simulink library "GFe_Lib"  (R2021a)
settings: Solver=VariableStepAuto  StartTime=0.0  StopTime=10.0  RelTol=1e-3
values from neighbouring files (symbols this model uses):
  Ki_i = 0    [Init_GFL.m]
  Kp_i = Lc_eq/wb*wn_i    [Init_GFL.m]
  Lf_pu = Lc_eq    [Init_GFL.m]
  Va0 = Vm0*sqrt(2)*Vb1*sin(Theta_Vm0*pi/180)    [Init_LF_L.m]    (also in Init_LF_MMC.m)
  Vb0 = Vm0*sqrt(2)*Vb1*sin(Theta_Vm0*pi/180-2*pi/3)    [Init_LF_L.m]    (also in Init_LF_MMC.m)
  Vc0 = Vm0*sqrt(2)*Vb1*sin(Theta_Vm0*pi/180+2*pi/3)    [Init_LF_L.m]    (also in Init_LF_MMC.m)
  Vm0_d = Vvsc0*cos(angle(Vvirt))    [Init_LF_L.m]    (also in Init_LF_MMC.m)
  Vm0_q = Vvsc0*sin(angle(Vvirt))    [Init_LF_L.m]    (also in Init_LF_MMC.m)
  Vvsc0 = abs(Vvirt)    [Init_LF_L.m]    (also in Init_LF_MMC.m)
undefined symbols (not defined in the file or in its folder): fb, Ib2, Sb, Solver_Time_Step, Time_Step, Vb1, Vb2, wb, Zb
libraries: Control_Lib x18, spsThreePhaseSourceLib x7, powerlib x7, spsThreePhaseBreakerLib x6, slpidlib x6, spsThreePhaseVIMeasurementLib x5, spsThreePhaseTransformerTwoWindingsLib x4, spsUniversalBridgeLib x3, spsVoltageMeasurementLib x3, spsRMSLib x2, spsDCVoltageSourceLib x2, spsSeriesRLCBranchLib x2
(part 3 of 3)

== system GFe_Lib/Mean Model 2-Level L-filter with DC Link/Control loops/ pu P//Q computation ==
  v_abc_pu : Inport  PortDimensions=3
  i_abc_pu : Inport  Port=2  PortDimensions=3
  Demux : Demux  Outputs=3
      settings: DisplayOption=none
  Mux : Mux  Inputs=3
  Product1 : Product  InputSameDT=on  SaturateOnIntegerOverflow=on  OutDataTypeStr=Inherit: Same as first input
  Product3 : Product  InputSameDT=on  SaturateOnIntegerOverflow=on  OutDataTypeStr=Inherit: Same as first input
  Sum : Sum  Inputs=+-  InputSameDT=on  SaturateOnIntegerOverflow=on  OutDataTypeStr=Inherit: Same as first input
  Sum1 : Sum  Inputs=1  InputSameDT=on  SaturateOnIntegerOverflow=on  OutDataTypeStr=Inherit: Same as first input
  Sum4 : Sum  Inputs=1  InputSameDT=on  SaturateOnIntegerOverflow=on  OutDataTypeStr=Inherit: Same as first input
  Sum5 : Sum  Inputs=+-  InputSameDT=on  SaturateOnIntegerOverflow=on  OutDataTypeStr=Inherit: Same as first input
  Sum6 : Sum  Inputs=+-  InputSameDT=on  SaturateOnIntegerOverflow=on  OutDataTypeStr=Inherit: Same as first input
  pu->V : Gain  Gain=1/sqrt(3)  SaturateOnIntegerOverflow=on  OutDataTypeStr=Inherit: Same as input  ParamDataTypeStr=Inherit: Same as input
  pu->V1 : Gain  Gain=1/3  SaturateOnIntegerOverflow=on  OutDataTypeStr=Inherit: Same as input  ParamDataTypeStr=Inherit: Same as input
  pu->V2 : Gain  Gain=1/3  SaturateOnIntegerOverflow=on  OutDataTypeStr=Inherit: Same as input  ParamDataTypeStr=Inherit: Same as input
  P : Outport  VectorParamsAs1DForOutWhenUnconnected=off
  Q : Outport  Port=2  VectorParamsAs1DForOutWhenUnconnected=off
  wires:
  pu->V/1 -> pu->V2/1  "Q"
  Mux/1 -> Product3/1
  Sum6/1 -> Mux/2
  Sum5/1 -> Mux/1
  Sum/1 -> Mux/3
  Demux/3 -> Sum6/1, Sum5/2
  Demux/2 -> Sum5/1, Sum/2
  Demux/1 -> Sum6/2, Sum/1
  Sum4/1 -> pu->V1/1
  i_abc_pu/1 -> Product3/2, Product1/2
  v_abc_pu/1 -> Demux/1, Product1/1
  Product1/1 -> Sum4/1
  Product3/1 -> Sum1/1
  Sum1/1 -> pu->V/1
  pu->V1/1 -> P/1
  pu->V2/1 -> Q/1

== system GFe_Lib/Mean Model 2-Level L-filter with DC Link/Control loops/Inner Current Control ==
  ig_dq_ref : Inport
  ig_dq : Inport  Port=2
  w_PLL : Inport  Port=3
  vg_dq : Inport  Port=4
  ig_dq_max : Inport  Port=5
  Current PI control : Subsystem
  vm_dq : Outport  VectorParamsAs1DForOutWhenUnconnected=off
  wires:
  w_PLL/1 -> Current PI control/4(w)  "w"
  vg_dq/1 -> Current PI control/2(Eg_dqfr)  "Eg_dq"
  ig_dq_ref/1 -> Current PI control/3(Is_dq_ref)
  Current PI control/1(vm_dq_ref) -> vm_dq/1  "vm_dq"
  ig_dq/1 -> Current PI control/1(Is_dq)  "Is_dq"
  ig_dq_max/1 -> Current PI control/5(Idq_ref_max)

== system GFe_Lib/Mean Model 2-Level L-filter with DC Link/Control loops/LPF ==
  In1 : Inport
  Add : Sum  Inputs=+-
  Gain : Gain  Gain=w_LPF
  Integrator : Integrator  InitialCondition=P0
  Out1 : Outport
  wires:
  In1/1 -> Add/1
  Integrator/1 -> Add/2, Out1/1
  Gain/1 -> Integrator/1
  Add/1 -> Gain/1

== system GFe_Lib/Mean Model 2-Level L-filter with DC Link/Control loops/LPF1 ==
  In1 : Inport
  Add : Sum  Inputs=+-
  Gain : Gain  Gain=w_LPF
  Integrator : Integrator  InitialCondition=V0
  Out1 : Outport
  wires:
  In1/1 -> Add/1
  Integrator/1 -> Add/2, Out1/1
  Gain/1 -> Integrator/1
  Add/1 -> Gain/1

== system GFe_Lib/Mean Model 2-Level L-filter with DC Link/Control loops/LPF2 ==
  In1 : Inport
  Add : Sum  Inputs=+-
  Gain : Gain  Gain=w_LPF
  Integrator : Integrator  InitialCondition=Q0
  Out1 : Outport
  wires:
  In1/1 -> Add/1
  Integrator/1 -> Add/2, Out1/1
  Gain/1 -> Integrator/1
  Add/1 -> Gain/1

== system GFe_Lib/Mean Model 2-Level L-filter with DC Link/Control loops/RMS derivation ==
  dq : Inport
  Demux : Demux  Outputs=2
  Sqrt : Sqrt  SaturateOnIntegerOverflow=on
  Square : Math  Operator=square  SaturateOnIntegerOverflow=on
  Square1 : Math  Operator=square  SaturateOnIntegerOverflow=on
  Sum : Sum
  rms : Outport
  wires:
  dq/1 -> Demux/1
  Demux/2 -> Square1/1
  Square/1 -> Sum/1
  Demux/1 -> Square/1
  Sqrt/1 -> rms/1
  Sum/1 -> Sqrt/1
  Square1/1 -> Sum/2

== system GFe_Lib/Mean Model 2-Level L-filter with DC Link/Control loops/norm1 ==
  In1 : Inport
  Add : Sum
  Demux : Demux  Outputs=2
  Sqrt : Sqrt  SaturateOnIntegerOverflow=on
  Square : Math  Operator=square  SaturateOnIntegerOverflow=on
  Square1 : Math  Operator=square  SaturateOnIntegerOverflow=on
  Out1 : Outport
  wires:
  In1/1 -> Demux/1
  Square1/1 -> Add/2
  Square/1 -> Add/1
  Demux/1 -> Square/1
  Demux/2 -> Square1/1
  Add/1 -> Sqrt/1
  Sqrt/1 -> Out1/1

== system GFe_Lib/Mean Model 2-Level L-filter with DC Link/Control loops/norm2 ==
  In1 : Inport
  Add : Sum
  Demux : Demux  Outputs=2
  Sqrt : Sqrt  SaturateOnIntegerOverflow=on
  Square : Math  Operator=square  SaturateOnIntegerOverflow=on
  Square1 : Math  Operator=square  SaturateOnIntegerOverflow=on
  Out1 : Outport
  wires:
  In1/1 -> Demux/1
  Square1/1 -> Add/2
  Square/1 -> Add/1
  Demux/1 -> Square/1
  Demux/2 -> Square1/1
  Add/1 -> Sqrt/1
  Sqrt/1 -> Out1/1

== system GFe_Lib/Mean Model 2-Level L-filter_sav/Control loops/ pu P//Q computation ==
  v_abc_pu : Inport  PortDimensions=3
  i_abc_pu : Inport  Port=2  PortDimensions=3
  Demux : Demux  Outputs=3
      settings: DisplayOption=none
  Mux : Mux  Inputs=3
  Product1 : Product  InputSameDT=on  SaturateOnIntegerOverflow=on  OutDataTypeStr=Inherit: Same as first input
  Product3 : Product  InputSameDT=on  SaturateOnIntegerOverflow=on  OutDataTypeStr=Inherit: Same as first input
  Sum : Sum  Inputs=+-  InputSameDT=on  SaturateOnIntegerOverflow=on  OutDataTypeStr=Inherit: Same as first input
  Sum1 : Sum  Inputs=1  InputSameDT=on  SaturateOnIntegerOverflow=on  OutDataTypeStr=Inherit: Same as first input
  Sum4 : Sum  Inputs=1  InputSameDT=on  SaturateOnIntegerOverflow=on  OutDataTypeStr=Inherit: Same as first input
  Sum5 : Sum  Inputs=+-  InputSameDT=on  SaturateOnIntegerOverflow=on  OutDataTypeStr=Inherit: Same as first input
  Sum6 : Sum  Inputs=+-  InputSameDT=on  SaturateOnIntegerOverflow=on  OutDataTypeStr=Inherit: Same as first input
  pu->V : Gain  Gain=1/sqrt(3)  SaturateOnIntegerOverflow=on  OutDataTypeStr=Inherit: Same as input  ParamDataTypeStr=Inherit: Same as input
  pu->V1 : Gain  Gain=1/3  SaturateOnIntegerOverflow=on  OutDataTypeStr=Inherit: Same as input  ParamDataTypeStr=Inherit: Same as input
  pu->V2 : Gain  Gain=1/3  SaturateOnIntegerOverflow=on  OutDataTypeStr=Inherit: Same as input  ParamDataTypeStr=Inherit: Same as input
  P : Outport  VectorParamsAs1DForOutWhenUnconnected=off
  Q : Outport  Port=2  VectorParamsAs1DForOutWhenUnconnected=off
  wires:
  pu->V2/1 -> Q/1
  pu->V1/1 -> P/1
  Sum1/1 -> pu->V/1
  Product3/1 -> Sum1/1
  Product1/1 -> Sum4/1
  v_abc_pu/1 -> Product1/1, Demux/1
  i_abc_pu/1 -> Product1/2, Product3/2
  Sum4/1 -> pu->V1/1
  Demux/1 -> Sum/1, Sum6/2
  Demux/2 -> Sum/2, Sum5/1
  Demux/3 -> Sum5/2, Sum6/1
  Sum/1 -> Mux/3
  Sum5/1 -> Mux/1
  Sum6/1 -> Mux/2
  Mux/1 -> Product3/1
  pu->V/1 -> pu->V2/1  "Q"

== system GFe_Lib/Mean Model 2-Level L-filter_sav/Control loops/Inner Current Control ==
  ig_dq_ref : Inport
  ig_dq : Inport  Port=2
  theta_PLL : Inport  Port=3
  w_PLL : Inport  Port=4
  vg_dq : Inport  Port=5
  Control Delay compensation : Constant  Value=wb*Solver_Time_Step
  Current PI control : Subsystem
  Mux : Mux  Inputs=2
  Sum : Sum  Inputs=|++
  Trigonometric Function : Trigonometry
  Trigonometric Function1 : Trigonometry  Operator=cos
  vm_dq : Outport  VectorParamsAs1DForOutWhenUnconnected=off
  CosSinTheta_delay : Outport  Port=2  VectorParamsAs1DForOutWhenUnconnected=off
  wires:
  ig_dq/1 -> Current PI control/1(Is_dq)  "Is_dq"
  Current PI control/1(vm_dq_ref) -> vm_dq/1  "vm_dq"
  ig_dq_ref/1 -> Current PI control/3(Is_dq_ref)
  vg_dq/1 -> Current PI control/2(Eg_dqfr)  "Eg_dq"
  w_PLL/1 -> Current PI control/4(w)  "w"
  Control Delay compensation/1 -> Sum/2
  Trigonometric Function/1 -> Mux/2
  Sum/1 -> Trigonometric Function/1, Trigonometric Function1/1
  theta_PLL/1 -> Sum/1  "Theta"
  Trigonometric Function1/1 -> Mux/1
  Mux/1 -> CosSinTheta_delay/1

== system GFe_Lib/Mean Model 2-Level LCL-filter [under construction]/Control loops/ pu P//Q computation ==
  v_abc_pu : Inport  PortDimensions=3
  i_abc_pu : Inport  Port=2  PortDimensions=3
  Demux : Demux  Outputs=3
      settings: DisplayOption=none
  Mux : Mux  Inputs=3
  Product1 : Product  InputSameDT=on  SaturateOnIntegerOverflow=on  OutDataTypeStr=Inherit: Same as first input
  Product3 : Product  InputSameDT=on  SaturateOnIntegerOverflow=on  OutDataTypeStr=Inherit: Same as first input
  Sum : Sum  Inputs=+-  InputSameDT=on  SaturateOnIntegerOverflow=on  OutDataTypeStr=Inherit: Same as first input
  Sum1 : Sum  Inputs=1  InputSameDT=on  SaturateOnIntegerOverflow=on  OutDataTypeStr=Inherit: Same as first input
  Sum4 : Sum  Inputs=1  InputSameDT=on  SaturateOnIntegerOverflow=on  OutDataTypeStr=Inherit: Same as first input
  Sum5 : Sum  Inputs=+-  InputSameDT=on  SaturateOnIntegerOverflow=on  OutDataTypeStr=Inherit: Same as first input
  Sum6 : Sum  Inputs=+-  InputSameDT=on  SaturateOnIntegerOverflow=on  OutDataTypeStr=Inherit: Same as first input
  pu->V : Gain  Gain=1/sqrt(3)  SaturateOnIntegerOverflow=on  OutDataTypeStr=Inherit: Same as input  ParamDataTypeStr=Inherit: Same as input
  pu->V1 : Gain  Gain=1/3  SaturateOnIntegerOverflow=on  OutDataTypeStr=Inherit: Same as input  ParamDataTypeStr=Inherit: Same as input
  pu->V2 : Gain  Gain=1/3  SaturateOnIntegerOverflow=on  OutDataTypeStr=Inherit: Same as input  ParamDataTypeStr=Inherit: Same as input
  P : Outport  VectorParamsAs1DForOutWhenUnconnected=off
  Q : Outport  Port=2  VectorParamsAs1DForOutWhenUnconnected=off
  wires:
  pu->V2/1 -> Q/1
  pu->V1/1 -> P/1
  Sum1/1 -> pu->V/1
  Product3/1 -> Sum1/1
  Product1/1 -> Sum4/1
  v_abc_pu/1 -> Product1/1, Demux/1
  i_abc_pu/1 -> Product1/2, Product3/2
  Sum4/1 -> pu->V1/1
  Demux/1 -> Sum/1, Sum6/2
  Demux/2 -> Sum/2, Sum5/1
  Demux/3 -> Sum5/2, Sum6/1
  Sum/1 -> Mux/3
  Sum5/1 -> Mux/1
  Sum6/1 -> Mux/2
  Mux/1 -> Product3/1
  pu->V/1 -> pu->V2/1  "Q"

== system GFe_Lib/Mean Model 2-Level LCL-filter [under construction]/Control loops/Inner Current Control ==
  ig_dq_ref : Inport
  ig_dq : Inport  Port=2
  theta_PLL : Inport  Port=3
  w_PLL : Inport  Port=4
  vg_dq : Inport  Port=5
  Current PI control : Subsystem
  vm_dq : Outport  VectorParamsAs1DForOutWhenUnconnected=off
  theta : Outport  Port=2  VectorParamsAs1DForOutWhenUnconnected=off
  wires:
  ig_dq/1 -> Current PI control/1(Is_dq)  "Is_dq"
  theta_PLL/1 -> theta/1  "Theta"
  Current PI control/1(vm_dq_ref) -> vm_dq/1  "vm_dq"
  ig_dq_ref/1 -> Current PI control/3(Is_dq_ref)
  vg_dq/1 -> Current PI control/2(Eg_dqfr)  "Eg_dq"
  w_PLL/1 -> Current PI control/4(w)  "w"

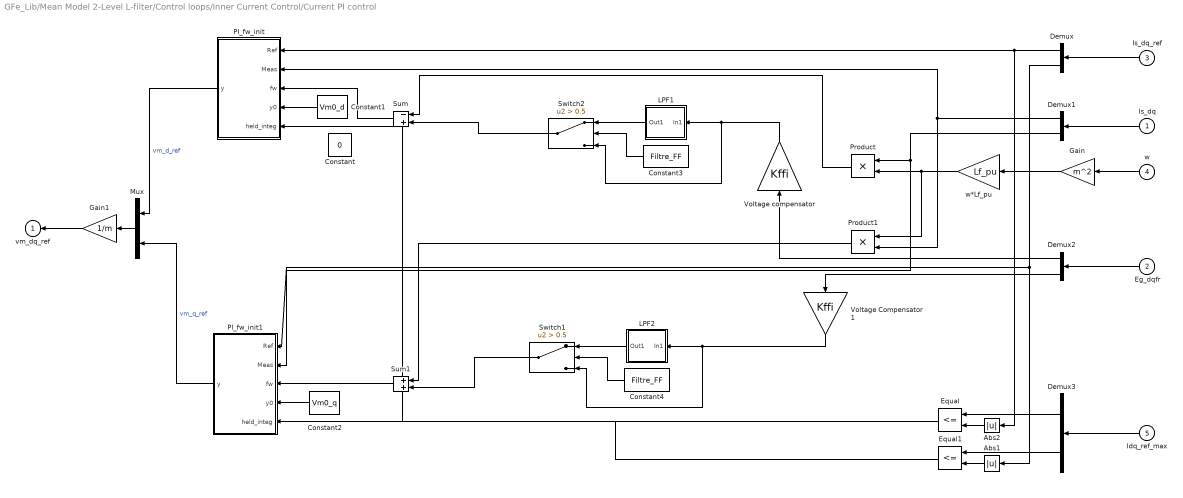
== system GFe_Lib/Mean Model 2-Level L-filter/Control loops/Inner Current Control/Current PI control ==
  Is_dq : Inport
  Eg_dqfr : Inport  Port=2
  Is_dq_ref : Inport  Port=3
  w : Inport  Port=4
  Idq_ref_max : Inport  Port=5
  Abs1 : Abs
  Abs2 : Abs
  Constant : Constant  Value=0
  Constant1 : Constant  Value=Vm0_d
  Constant2 : Constant  Value=Vm0_q
  Constant3 : Constant  Value=Filtre_FF
  Constant4 : Constant  Value=Filtre_FF
  Demux{,1..3} (4 alike) : Demux  Outputs=2
  Equal : RelationalOperator  Operator=<=  OutDataTypeStr=boolean  RndMeth=Simplest
  Equal1 : RelationalOperator  Operator=<=  OutDataTypeStr=boolean  RndMeth=Simplest
  Gain : Gain  Gain=m^2
  Gain1 : Gain  Gain=1/m
  LPF1 : Subsystem
  LPF2 : Subsystem
  Mux : Mux  Inputs=[1 1]
  PI_fw_init : Subsystem  AncestorBlock=Control_Lib/PI_fw_init  TreatAsAtomicUnit=on  mask{Kp=Kp_i, Ki=Ki_i}
  PI_fw_init1 : Subsystem  AncestorBlock=Control_Lib/PI_fw_init  TreatAsAtomicUnit=on  mask{Kp=Kp_i, Ki=Ki_i}
  Product : Product  RndMeth=Zero
  Product1 : Product  RndMeth=Zero
  Sum : Sum  Inputs=-+
  Sum1 : Sum
  Switch1 : Switch  Criteria=u2 > Threshold  Threshold=0.5
  Switch2 : Switch  Criteria=u2 > Threshold  Threshold=0.5
  Voltage Compensator 1 : Gain  Gain=Kffi
  Voltage compensator : Gain  Gain=Kffi
  w*Lf_pu : Gain  Gain=Lf_pu
  vm_dq_ref : Outport  InitialOutput=0  VectorParamsAs1DForOutWhenUnconnected=off
  wires:
  Voltage compensator/1 -> Switch2/3, LPF1/1(In1)
  w/1 -> Gain/1
  PI_fw_init1/1(y) -> Mux/2  "vm_q_ref"
  PI_fw_init/1(y) -> Mux/1  "vm_d_ref"
  Product1/1 -> Sum1/1
  Demux/2 -> Abs1/1, PI_fw_init1/1(Ref)
  Mux/1 -> Gain1/1
  Demux1/2 -> PI_fw_init1/2(Meas), Product/1
  w*Lf_pu/1 -> Product/2, Product1/1
  Demux1/1 -> PI_fw_init/2(Meas), Product1/2
  Demux/1 -> PI_fw_init/1(Ref), Abs2/1
  Is_dq_ref/1 -> Demux/1
  Is_dq/1 -> Demux1/1
  Eg_dqfr/1 -> Demux2/1
  Product/1 -> Sum/1
  Sum/1 -> PI_fw_init/3(fw)
  Constant1/1 -> PI_fw_init/4(y0)
  Sum1/1 -> PI_fw_init1/3(fw)
  Constant2/1 -> PI_fw_init1/4(y0)
  Demux2/1 -> Voltage compensator/1
  Demux2/2 -> Voltage Compensator 1/1
  Idq_ref_max/1 -> Demux3/1
  Demux3/1 -> Equal/1
  Demux3/2 -> Equal1/1
  Abs2/1 -> Equal/2
  Abs1/1 -> Equal1/2
  Equal/1 -> PI_fw_init/5(held_integ)
  Equal1/1 -> PI_fw_init1/5(held_integ)
  Gain/1 -> w*Lf_pu/1
  Gain1/1 -> vm_dq_ref/1
  LPF1/1(Out1) -> Switch2/1
  Constant3/1 -> Switch2/2
  Switch2/1 -> Sum/2
  LPF2/1(Out1) -> Switch1/1
  Voltage Compensator 1/1 -> Switch1/3, LPF2/1(In1)
  Constant4/1 -> Switch1/2
  Switch1/1 -> Sum1/2

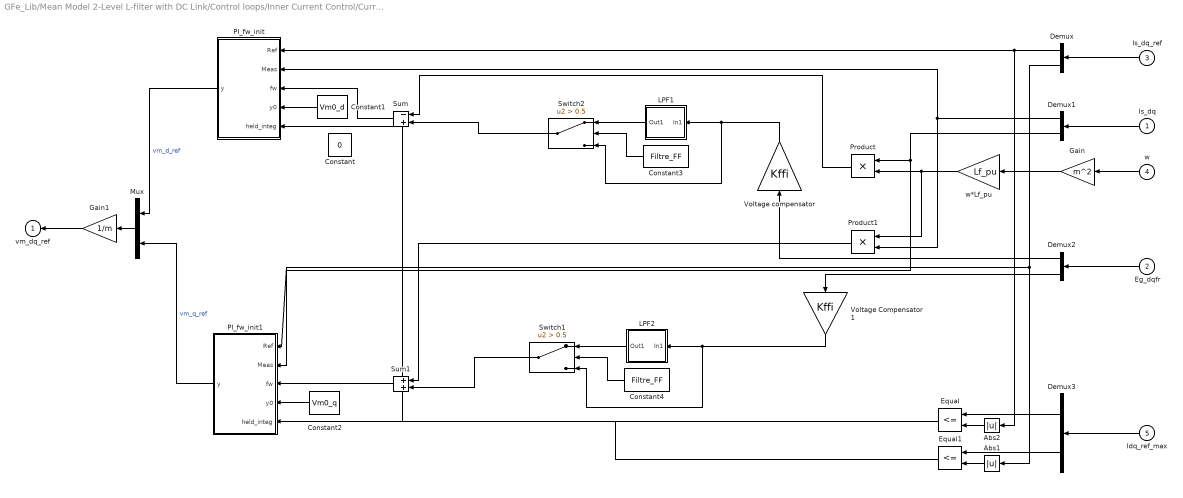
== system GFe_Lib/Mean Model 2-Level L-filter with DC Link/Control loops/Inner Current Control/Current PI control ==
  Is_dq : Inport
  Eg_dqfr : Inport  Port=2
  Is_dq_ref : Inport  Port=3
  w : Inport  Port=4
  Idq_ref_max : Inport  Port=5
  Abs1 : Abs
  Abs2 : Abs
  Constant : Constant  Value=0
  Constant1 : Constant  Value=Vm0_d
  Constant2 : Constant  Value=Vm0_q
  Constant3 : Constant  Value=Filtre_FF
  Constant4 : Constant  Value=Filtre_FF
  Demux{,1..3} (4 alike) : Demux  Outputs=2
  Equal : RelationalOperator  Operator=<=  OutDataTypeStr=boolean  RndMeth=Simplest
  Equal1 : RelationalOperator  Operator=<=  OutDataTypeStr=boolean  RndMeth=Simplest
  Gain : Gain  Gain=m^2
  Gain1 : Gain  Gain=1/m
  LPF1 : Subsystem
  LPF2 : Subsystem
  Mux : Mux  Inputs=[1 1]
  PI_fw_init : Subsystem  AncestorBlock=Control_Lib/PI_fw_init  TreatAsAtomicUnit=on  mask{Kp=Kp_i, Ki=Ki_i}
  PI_fw_init1 : Subsystem  AncestorBlock=Control_Lib/PI_fw_init  TreatAsAtomicUnit=on  mask{Kp=Kp_i, Ki=Ki_i}
  Product : Product  RndMeth=Zero
  Product1 : Product  RndMeth=Zero
  Sum : Sum  Inputs=-+
  Sum1 : Sum
  Switch1 : Switch  Criteria=u2 > Threshold  Threshold=0.5
  Switch2 : Switch  Criteria=u2 > Threshold  Threshold=0.5
  Voltage Compensator 1 : Gain  Gain=Kffi
  Voltage compensator : Gain  Gain=Kffi
  w*Lf_pu : Gain  Gain=Lf_pu
  vm_dq_ref : Outport  InitialOutput=0  VectorParamsAs1DForOutWhenUnconnected=off
  wires:
  Voltage compensator/1 -> Switch2/3, LPF1/1(In1)
  w/1 -> Gain/1
  PI_fw_init1/1(y) -> Mux/2  "vm_q_ref"
  PI_fw_init/1(y) -> Mux/1  "vm_d_ref"
  Product1/1 -> Sum1/1
  Demux/2 -> Abs1/1, PI_fw_init1/1(Ref)
  Mux/1 -> Gain1/1
  Demux1/2 -> PI_fw_init1/2(Meas), Product/1
  w*Lf_pu/1 -> Product/2, Product1/1
  Demux1/1 -> PI_fw_init/2(Meas), Product1/2
  Demux/1 -> PI_fw_init/1(Ref), Abs2/1
  Is_dq_ref/1 -> Demux/1
  Is_dq/1 -> Demux1/1
  Eg_dqfr/1 -> Demux2/1
  Product/1 -> Sum/1
  Sum/1 -> PI_fw_init/3(fw)
  Constant1/1 -> PI_fw_init/4(y0)
  Sum1/1 -> PI_fw_init1/3(fw)
  Constant2/1 -> PI_fw_init1/4(y0)
  Demux2/1 -> Voltage compensator/1
  Demux2/2 -> Voltage Compensator 1/1
  Idq_ref_max/1 -> Demux3/1
  Demux3/1 -> Equal/1
  Demux3/2 -> Equal1/1
  Abs2/1 -> Equal/2
  Abs1/1 -> Equal1/2
  Equal/1 -> PI_fw_init/5(held_integ)
  Equal1/1 -> PI_fw_init1/5(held_integ)
  Gain/1 -> w*Lf_pu/1
  Gain1/1 -> vm_dq_ref/1
  LPF1/1(Out1) -> Switch2/1
  Constant3/1 -> Switch2/2
  Switch2/1 -> Sum/2
  LPF2/1(Out1) -> Switch1/1
  Voltage Compensator 1/1 -> Switch1/3, LPF2/1(In1)
  Constant4/1 -> Switch1/2
  Switch1/1 -> Sum1/2

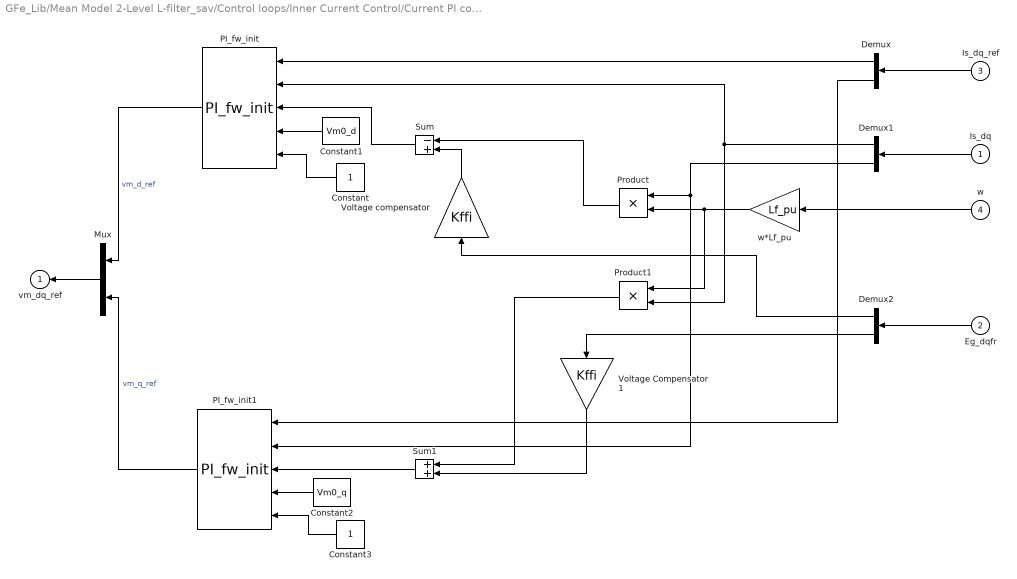
== system GFe_Lib/Mean Model 2-Level L-filter_sav/Control loops/Inner Current Control/Current PI control ==
  Is_dq : Inport
  Eg_dqfr : Inport  Port=2
  Is_dq_ref : Inport  Port=3
  w : Inport  Port=4
  Constant : Constant
  Constant1 : Constant  Value=Vm0_d
  Constant2 : Constant  Value=Vm0_q
  Constant3 : Constant
  Demux : Demux  Outputs=2
  Demux1 : Demux  Outputs=2
  Demux2 : Demux  Outputs=2
  Mux : Mux  Inputs=[1 1]
  PI_fw_init : Control_Lib/PI_fw_init  Kp=Kp_i  Ki=Ki_i
      settings: SourceProductName=VSC4SPS
  PI_fw_init1 : Control_Lib/PI_fw_init  Kp=Kp_i  Ki=Ki_i
      settings: SourceProductName=VSC4SPS
  Product : Product  RndMeth=Zero
  Product1 : Product  RndMeth=Zero
  Sum : Sum  Inputs=-+
  Sum1 : Sum
  Voltage Compensator 1 : Gain  Gain=Kffi
  Voltage compensator : Gain  Gain=Kffi
  w*Lf_pu : Gain  Gain=Lf_pu
  vm_dq_ref : Outport  InitialOutput=0  VectorParamsAs1DForOutWhenUnconnected=off
  wires:
  Constant3/1 -> PI_fw_init1/5
  Constant2/1 -> PI_fw_init1/4
  Voltage Compensator 1/1 -> Sum1/2
  Sum1/1 -> PI_fw_init1/3
  Constant1/1 -> PI_fw_init/4
  Constant/1 -> PI_fw_init/5
  Sum/1 -> PI_fw_init/3
  Product/1 -> Sum/1
  Eg_dqfr/1 -> Demux2/1
  Demux2/2 -> Voltage Compensator 1/1
  Demux2/1 -> Voltage compensator/1
  Is_dq/1 -> Demux1/1
  Is_dq_ref/1 -> Demux/1
  Demux/1 -> PI_fw_init/1
  Demux1/1 -> Product1/2, PI_fw_init/2
  w*Lf_pu/1 -> Product1/1, Product/2
  Demux1/2 -> Product/1, PI_fw_init1/2
  Mux/1 -> vm_dq_ref/1
  Demux/2 -> PI_fw_init1/1
  Product1/1 -> Sum1/1
  PI_fw_init/1 -> Mux/1  "vm_d_ref"
  PI_fw_init1/1 -> Mux/2  "vm_q_ref"
  w/1 -> w*Lf_pu/1
  Voltage compensator/1 -> Sum/2

== system GFe_Lib/Mean Model 2-Level LCL-filter [under construction]/Control loops/Inner Current Control/Current PI control ==
  Is_dq : Inport
  Eg_dqfr : Inport  Port=2
  Is_dq_ref : Inport  Port=3
  w : Inport  Port=4
  Constant : Constant
  Constant1 : Constant  Value=Vm0_d
  Constant2 : Constant  Value=Vm0_q
  Constant3 : Constant
  Demux : Demux  Outputs=2
  Demux1 : Demux  Outputs=2
  Demux2 : Demux  Outputs=2
  Mux : Mux  Inputs=[1 1]
  PI_fw_init : Control_Lib/PI_fw_init  Kp=Kp_i  Ki=Ki_i
      settings: SourceProductName=VSC4SPS
  PI_fw_init1 : Control_Lib/PI_fw_init  Kp=Kp_i  Ki=Ki_i
      settings: SourceProductName=VSC4SPS
  Product : Product  RndMeth=Zero
  Product1 : Product  RndMeth=Zero
  Sum : Sum  Inputs=-+
  Sum1 : Sum
  Voltage Compensator 1 : Gain  Gain=Kffi
  Voltage compensator : Gain  Gain=Kffi
  w*Lf_pu : Gain  Gain=Lf_pu
  vm_dq_ref : Outport  InitialOutput=0  VectorParamsAs1DForOutWhenUnconnected=off
  wires:
  Constant3/1 -> PI_fw_init1/5
  Constant2/1 -> PI_fw_init1/4
  Voltage Compensator 1/1 -> Sum1/2
  Sum1/1 -> PI_fw_init1/3
  Constant1/1 -> PI_fw_init/4
  Constant/1 -> PI_fw_init/5
  Sum/1 -> PI_fw_init/3
  Product/1 -> Sum/1
  Eg_dqfr/1 -> Demux2/1
  Demux2/2 -> Voltage Compensator 1/1
  Demux2/1 -> Voltage compensator/1
  Is_dq/1 -> Demux1/1
  Is_dq_ref/1 -> Demux/1
  Demux/1 -> PI_fw_init/1
  Demux1/1 -> Product1/2, PI_fw_init/2
  w*Lf_pu/1 -> Product1/1, Product/2
  Demux1/2 -> Product/1, PI_fw_init1/2
  Mux/1 -> vm_dq_ref/1
  Demux/2 -> PI_fw_init1/1
  Product1/1 -> Sum1/1
  PI_fw_init/1 -> Mux/1  "vm_d_ref"
  PI_fw_init1/1 -> Mux/2  "vm_q_ref"
  w/1 -> w*Lf_pu/1
  Voltage compensator/1 -> Sum/2

== system GFe_Lib/Mean Model 2-Level L-filter/Control loops/Inner Current Control/Current PI control/LPF1 ==
  In1 : Inport
  Add : Sum  Inputs=+-
  Gain : Gain  Gain=w_ff
  Integrator : Integrator  InitialCondition=V0*cos(Theta0*pi/180)
  Out1 : Outport
  wires:
  In1/1 -> Add/1
  Integrator/1 -> Add/2, Out1/1
  Gain/1 -> Integrator/1
  Add/1 -> Gain/1

== system GFe_Lib/Mean Model 2-Level L-filter/Control loops/Inner Current Control/Current PI control/LPF2 ==
  In1 : Inport
  Add : Sum  Inputs=+-
  Gain : Gain  Gain=w_ff
  Integrator : Integrator  InitialCondition=V0*sin(Theta0*pi/180)
  Out1 : Outport
  wires:
  In1/1 -> Add/1
  Integrator/1 -> Add/2, Out1/1
  Gain/1 -> Integrator/1
  Add/1 -> Gain/1

== system GFe_Lib/Mean Model 2-Level L-filter/Control loops/Inner Current Control/Current PI control/PI_fw_init ==
  Ref : Inport
  Meas : Inport  Port=2
  fw : Inport  Port=3
  y0 : Inport  Port=4
  held_integ : Inport  Port=5
  Constant : Constant  Value=0
  Constant1 : Constant  Value=0
  Data Type Conversion : DataTypeConversion
  Gain : Gain  Gain=Kp
  Gain1 : Gain  Gain=Ki
  Init_condition : Subsystem
  Integrator : Integrator  InitialConditionSource=external
  Memory : Memory  InitialCondition=1
  Subsystem : Subsystem  Commented=on
  Sum : Sum
  Sum1 : Sum  Inputs=+-
  Sum2 : Sum
  Switch : Switch  Criteria=u2 > Threshold  Threshold=0.5
  y : Outport  VectorParamsAs1DForOutWhenUnconnected=off
  wires:
  Init_condition/1(integ0) -> Integrator/2
  [comp] -> Init_condition/2(comp)
  Ref/1 -> Sum1/1
  Meas/1 -> Sum1/2
  Sum/1 -> Sum2/1, [comp]
  Sum1/1 -> Gain/1, Gain1/1
  Sum2/1 -> y/1
  y0/1 -> Init_condition/1(y0)
  Constant/1 -> Memory/1
  Memory/1 -> Init_condition/Enable
  fw/1 -> Sum/1
  Gain/1 -> Sum/2
  Integrator/1 -> Sum2/2
  Switch/1 -> Integrator/1
  Constant1/1 -> Switch/1
  Gain1/1 -> Switch/3
  held_integ/1 -> Data Type Conversion/1
  Data Type Conversion/1 -> Switch/2

== system GFe_Lib/Mean Model 2-Level L-filter/Control loops/Inner Current Control/Current PI control/PI_fw_init1 ==
  Ref : Inport
  Meas : Inport  Port=2
  fw : Inport  Port=3
  y0 : Inport  Port=4
  held_integ : Inport  Port=5
  Constant : Constant  Value=0
  Constant1 : Constant  Value=0
  Data Type Conversion : DataTypeConversion
  Gain : Gain  Gain=Kp
  Gain1 : Gain  Gain=Ki
  Init_condition : Subsystem
  Integrator : Integrator  InitialConditionSource=external
  Memory : Memory  InitialCondition=1
  Subsystem : Subsystem  Commented=on
  Sum : Sum
  Sum1 : Sum  Inputs=+-
  Sum2 : Sum
  Switch : Switch  Criteria=u2 > Threshold  Threshold=0.5
  y : Outport  VectorParamsAs1DForOutWhenUnconnected=off
  wires:
  Init_condition/1(integ0) -> Integrator/2
  [comp] -> Init_condition/2(comp)
  Ref/1 -> Sum1/1
  Meas/1 -> Sum1/2
  Sum/1 -> Sum2/1, [comp]
  Sum1/1 -> Gain/1, Gain1/1
  Sum2/1 -> y/1
  y0/1 -> Init_condition/1(y0)
  Constant/1 -> Memory/1
  Memory/1 -> Init_condition/Enable
  fw/1 -> Sum/1
  Gain/1 -> Sum/2
  Integrator/1 -> Sum2/2
  Switch/1 -> Integrator/1
  Constant1/1 -> Switch/1
  Gain1/1 -> Switch/3
  held_integ/1 -> Data Type Conversion/1
  Data Type Conversion/1 -> Switch/2

== system GFe_Lib/Mean Model 2-Level L-filter with DC Link/Control loops/Inner Current Control/Current PI control/LPF1 ==
  In1 : Inport
  Add : Sum  Inputs=+-
  Gain : Gain  Gain=w_ff
  Integrator : Integrator  InitialCondition=V0*cos(Theta0*pi/180)
  Out1 : Outport
  wires:
  In1/1 -> Add/1
  Integrator/1 -> Add/2, Out1/1
  Gain/1 -> Integrator/1
  Add/1 -> Gain/1

== system GFe_Lib/Mean Model 2-Level L-filter with DC Link/Control loops/Inner Current Control/Current PI control/LPF2 ==
  In1 : Inport
  Add : Sum  Inputs=+-
  Gain : Gain  Gain=w_ff
  Integrator : Integrator  InitialCondition=V0*sin(Theta0*pi/180)
  Out1 : Outport
  wires:
  In1/1 -> Add/1
  Integrator/1 -> Add/2, Out1/1
  Gain/1 -> Integrator/1
  Add/1 -> Gain/1

== system GFe_Lib/Mean Model 2-Level L-filter with DC Link/Control loops/Inner Current Control/Current PI control/PI_fw_init ==
  Ref : Inport
  Meas : Inport  Port=2
  fw : Inport  Port=3
  y0 : Inport  Port=4
  held_integ : Inport  Port=5
  Constant : Constant  Value=0
  Constant1 : Constant  Value=0
  Data Type Conversion : DataTypeConversion
  Gain : Gain  Gain=Kp
  Gain1 : Gain  Gain=Ki
  Init_condition : Subsystem
  Integrator : Integrator  InitialConditionSource=external
  Memory : Memory  InitialCondition=1
  Subsystem : Subsystem  Commented=on
  Sum : Sum
  Sum1 : Sum  Inputs=+-
  Sum2 : Sum
  Switch : Switch  Criteria=u2 > Threshold  Threshold=0.5
  y : Outport  VectorParamsAs1DForOutWhenUnconnected=off
  wires:
  Init_condition/1(integ0) -> Integrator/2
  [comp] -> Init_condition/2(comp)
  Ref/1 -> Sum1/1
  Meas/1 -> Sum1/2
  Sum/1 -> Sum2/1, [comp]
  Sum1/1 -> Gain/1, Gain1/1
  Sum2/1 -> y/1
  y0/1 -> Init_condition/1(y0)
  Constant/1 -> Memory/1
  Memory/1 -> Init_condition/Enable
  fw/1 -> Sum/1
  Gain/1 -> Sum/2
  Integrator/1 -> Sum2/2
  Switch/1 -> Integrator/1
  Constant1/1 -> Switch/1
  Gain1/1 -> Switch/3
  held_integ/1 -> Data Type Conversion/1
  Data Type Conversion/1 -> Switch/2

== system GFe_Lib/Mean Model 2-Level L-filter with DC Link/Control loops/Inner Current Control/Current PI control/PI_fw_init1 ==
  Ref : Inport
  Meas : Inport  Port=2
  fw : Inport  Port=3
  y0 : Inport  Port=4
  held_integ : Inport  Port=5
  Constant : Constant  Value=0
  Constant1 : Constant  Value=0
  Data Type Conversion : DataTypeConversion
  Gain : Gain  Gain=Kp
  Gain1 : Gain  Gain=Ki
  Init_condition : Subsystem
  Integrator : Integrator  InitialConditionSource=external
  Memory : Memory  InitialCondition=1
  Subsystem : Subsystem  Commented=on
  Sum : Sum
  Sum1 : Sum  Inputs=+-
  Sum2 : Sum
  Switch : Switch  Criteria=u2 > Threshold  Threshold=0.5
  y : Outport  VectorParamsAs1DForOutWhenUnconnected=off
  wires:
  Init_condition/1(integ0) -> Integrator/2
  [comp] -> Init_condition/2(comp)
  Ref/1 -> Sum1/1
  Meas/1 -> Sum1/2
  Sum/1 -> Sum2/1, [comp]
  Sum1/1 -> Gain/1, Gain1/1
  Sum2/1 -> y/1
  y0/1 -> Init_condition/1(y0)
  Constant/1 -> Memory/1
  Memory/1 -> Init_condition/Enable
  fw/1 -> Sum/1
  Gain/1 -> Sum/2
  Integrator/1 -> Sum2/2
  Switch/1 -> Integrator/1
  Constant1/1 -> Switch/1
  Gain1/1 -> Switch/3
  held_integ/1 -> Data Type Conversion/1
  Data Type Conversion/1 -> Switch/2

== system GFe_Lib/Mean Model 2-Level L-filter/Control loops/Inner Current Control/Current PI control/PI_fw_init/Init_condition ==
  y0 : Inport
  comp : Inport  Port=2
  Enable : EnablePort
  Sum : Sum  Inputs=-+
  integ0 : Outport  VectorParamsAs1DForOutWhenUnconnected=off
  wires:
  Sum/1 -> integ0/1
  y0/1 -> Sum/2
  comp/1 -> Sum/1

== system GFe_Lib/Mean Model 2-Level L-filter/Control loops/Inner Current Control/Current PI control/PI_fw_init/Subsystem ==
  e : Inport
  x0 : Inport  Port=2
  Enable : EnablePort
  Integrator : Integrator  InitialConditionSource=external
  y : Outport  VectorParamsAs1DForOutWhenUnconnected=off
  wires:
  x0/1 -> Integrator/2
  Integrator/1 -> y/1
  e/1 -> Integrator/1

== system GFe_Lib/Mean Model 2-Level L-filter/Control loops/Inner Current Control/Current PI control/PI_fw_init1/Init_condition ==
  y0 : Inport
  comp : Inport  Port=2
  Enable : EnablePort
  Sum : Sum  Inputs=-+
  integ0 : Outport  VectorParamsAs1DForOutWhenUnconnected=off
  wires:
  Sum/1 -> integ0/1
  y0/1 -> Sum/2
  comp/1 -> Sum/1

== system GFe_Lib/Mean Model 2-Level L-filter/Control loops/Inner Current Control/Current PI control/PI_fw_init1/Subsystem ==
  e : Inport
  x0 : Inport  Port=2
  Enable : EnablePort
  Integrator : Integrator  InitialConditionSource=external
  y : Outport  VectorParamsAs1DForOutWhenUnconnected=off
  wires:
  x0/1 -> Integrator/2
  Integrator/1 -> y/1
  e/1 -> Integrator/1

== system GFe_Lib/Mean Model 2-Level L-filter with DC Link/Control loops/Inner Current Control/Current PI control/PI_fw_init/Init_condition ==
  y0 : Inport
  comp : Inport  Port=2
  Enable : EnablePort
  Sum : Sum  Inputs=-+
  integ0 : Outport  VectorParamsAs1DForOutWhenUnconnected=off
  wires:
  Sum/1 -> integ0/1
  y0/1 -> Sum/2
  comp/1 -> Sum/1

== system GFe_Lib/Mean Model 2-Level L-filter with DC Link/Control loops/Inner Current Control/Current PI control/PI_fw_init/Subsystem ==
  e : Inport
  x0 : Inport  Port=2
  Enable : EnablePort
  Integrator : Integrator  InitialConditionSource=external
  y : Outport  VectorParamsAs1DForOutWhenUnconnected=off
  wires:
  x0/1 -> Integrator/2
  Integrator/1 -> y/1
  e/1 -> Integrator/1

== system GFe_Lib/Mean Model 2-Level L-filter with DC Link/Control loops/Inner Current Control/Current PI control/PI_fw_init1/Init_condition ==
  y0 : Inport
  comp : Inport  Port=2
  Enable : EnablePort
  Sum : Sum  Inputs=-+
  integ0 : Outport  VectorParamsAs1DForOutWhenUnconnected=off
  wires:
  Sum/1 -> integ0/1
  y0/1 -> Sum/2
  comp/1 -> Sum/1

== system GFe_Lib/Mean Model 2-Level L-filter with DC Link/Control loops/Inner Current Control/Current PI control/PI_fw_init1/Subsystem ==
  e : Inport
  x0 : Inport  Port=2
  Enable : EnablePort
  Integrator : Integrator  InitialConditionSource=external
  y : Outport  VectorParamsAs1DForOutWhenUnconnected=off
  wires:
  x0/1 -> Integrator/2
  Integrator/1 -> y/1
  e/1 -> Integrator/1
